simulink library "NMEA"  (R2024a)
settings: Solver=VariableStepAuto  StartTime=0.0  StopTime=10.0  RelTol=1e-3
libraries: $bdroot x44, simulink x21, simulink_extras x17, etargetslib x14
(part 3 of 4)

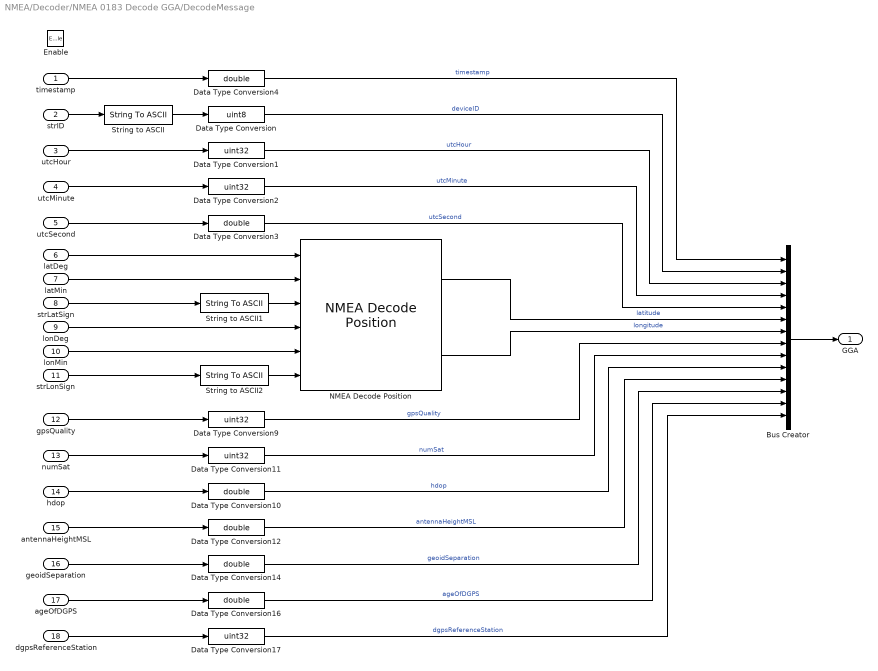
== system NMEA/Decoder/NMEA 0183 Decode GGA/DecodeMessage ==
  timestamp : Inport
  strID : Inport  Port=2
  utcHour : Inport  Port=3
  utcMinute : Inport  Port=4
  utcSecond : Inport  Port=5
  latDeg : Inport  Port=6
  latMin : Inport  Port=7
  strLatSign : Inport  Port=8
  lonDeg : Inport  Port=9
  lonMin : Inport  Port=10
  strLonSign : Inport  Port=11
  gpsQuality : Inport  Port=12
  numSat : Inport  Port=13
  hdop : Inport  Port=14
  antennaHeightMSL : Inport  Port=15
  geoidSeparation : Inport  Port=16
  ageOfDGPS : Inport  Port=17
  dgpsReferenceStation : Inport  Port=18
  Enable : EnablePort
  Bus Creator : BusCreator  Inputs=14
  Data Type Conversion : DataTypeConversion  OutDataTypeStr=uint8  SaturateOnIntegerOverflow=off  RndMeth=Floor
  Data Type Conversion{1..2,9,11,17} (5 alike) : DataTypeConversion  OutDataTypeStr=uint32  SaturateOnIntegerOverflow=off  RndMeth=Floor
  Data Type Conversion{3..4,10,12,14,16} (6 alike) : DataTypeConversion  OutDataTypeStr=double  SaturateOnIntegerOverflow=off  RndMeth=Floor
  NMEA Decode Position : $bdroot/Details/NMEA Decode Position
  String to ASCII : StringToASCII  OutputVectorSize=2
  String to ASCII1 : StringToASCII  OutputVectorSize=1
  String to ASCII2 : StringToASCII  OutputVectorSize=1
  GGA : Outport
  wires:
  Bus Creator/1 -> GGA/1
  timestamp/1 -> Data Type Conversion4/1
  strID/1 -> String to ASCII/1
  String to ASCII/1 -> Data Type Conversion/1
  Data Type Conversion/1 -> Bus Creator/2  "deviceID"
  utcHour/1 -> Data Type Conversion1/1
  utcMinute/1 -> Data Type Conversion2/1
  utcSecond/1 -> Data Type Conversion3/1
  Data Type Conversion1/1 -> Bus Creator/3  "utcHour"
  Data Type Conversion2/1 -> Bus Creator/4  "utcMinute"
  Data Type Conversion3/1 -> Bus Creator/5  "utcSecond"
  Data Type Conversion4/1 -> Bus Creator/1  "timestamp"
  gpsQuality/1 -> Data Type Conversion9/1
  numSat/1 -> Data Type Conversion11/1
  hdop/1 -> Data Type Conversion10/1
  antennaHeightMSL/1 -> Data Type Conversion12/1
  geoidSeparation/1 -> Data Type Conversion14/1
  ageOfDGPS/1 -> Data Type Conversion16/1
  dgpsReferenceStation/1 -> Data Type Conversion17/1
  Data Type Conversion9/1 -> Bus Creator/8  "gpsQuality"
  Data Type Conversion11/1 -> Bus Creator/9  "numSat"
  Data Type Conversion10/1 -> Bus Creator/10  "hdop"
  Data Type Conversion12/1 -> Bus Creator/11  "antennaHeightMSL"
  Data Type Conversion14/1 -> Bus Creator/12  "geoidSeparation"
  Data Type Conversion16/1 -> Bus Creator/13  "ageOfDGPS"
  Data Type Conversion17/1 -> Bus Creator/14  "dgpsReferenceStation"
  strLonSign/1 -> String to ASCII2/1
  String to ASCII1/1 -> NMEA Decode Position/3
  strLatSign/1 -> String to ASCII1/1
  String to ASCII2/1 -> NMEA Decode Position/6
  lonMin/1 -> NMEA Decode Position/5
  lonDeg/1 -> NMEA Decode Position/4
  latMin/1 -> NMEA Decode Position/2
  latDeg/1 -> NMEA Decode Position/1
  NMEA Decode Position/2 -> Bus Creator/7  "longitude"
  NMEA Decode Position/1 -> Bus Creator/6  "latitude"

== system NMEA/Decoder/NMEA 0183 Decode HDT/DecodeMessage ==
  timestamp : Inport
  strID : Inport  Port=2
  trueHeading : Inport  Port=3
  Enable : EnablePort
  Bus Creator : BusCreator  Inputs=3
  Data Type Conversion : DataTypeConversion  OutDataTypeStr=uint8  SaturateOnIntegerOverflow=off  RndMeth=Floor
  Data Type Conversion1 : DataTypeConversion  OutDataTypeStr=double  SaturateOnIntegerOverflow=off  RndMeth=Floor
  Data Type Conversion4 : DataTypeConversion  OutDataTypeStr=double  SaturateOnIntegerOverflow=off  RndMeth=Floor
  Degrees to Radians : simulink_extras/Transformations/Degrees to Radians
  Ensure Symmetrical Angle : $bdroot/Details/Ensure Symmetrical Angle
  String to ASCII : StringToASCII  OutputVectorSize=2
  HDT : Outport
  wires:
  Bus Creator/1 -> HDT/1
  Data Type Conversion/1 -> Bus Creator/2  "deviceID"
  Data Type Conversion4/1 -> Bus Creator/1  "timestamp"
  timestamp/1 -> Data Type Conversion4/1
  strID/1 -> String to ASCII/1
  String to ASCII/1 -> Data Type Conversion/1
  trueHeading/1 -> Data Type Conversion1/1
  Data Type Conversion1/1 -> Degrees to Radians/1
  Ensure Symmetrical Angle/1 -> Bus Creator/3  "trueHeading"
  Degrees to Radians/1 -> Ensure Symmetrical Angle/1

== system NMEA/Decoder/NMEA 0183 Decode MDA/DecodeMessage ==
  timestamp : Inport
  strID : Inport  Port=2
  pressureBar : Inport  Port=3
  airTemperatureC : Inport  Port=4
  Enable : EnablePort
  BarToPascal : Gain  Gain=1e5
  Bus Creator : BusCreator  Inputs=4
  String to ASCII : StringToASCII  OutputVectorSize=2
  MDA : Outport
  wires:
  strID/1 -> String to ASCII/1
  pressureBar/1 -> BarToPascal/1
  timestamp/1 -> Bus Creator/1  "timestamp"
  String to ASCII/1 -> Bus Creator/2  "deviceID"
  BarToPascal/1 -> Bus Creator/3  "pressure"
  airTemperatureC/1 -> Bus Creator/4  "airTemperature"
  Bus Creator/1 -> MDA/1

== system NMEA/Decoder/NMEA 0183 Decode MWV/DecodeMessage ==
  timestamp : Inport
  strID : Inport  Port=2
  windAngle : Inport  Port=3
  strWindAngleReference : Inport  Port=4
  windSpeed : Inport  Port=5
  strWindSpeedUnit : Inport  Port=6
  strStatus : Inport  Port=7
  Enable : EnablePort
  Bus Creator : BusCreator  Inputs=6
  Data Type Conversion{,2..3,5} (4 alike) : DataTypeConversion  OutDataTypeStr=uint8  SaturateOnIntegerOverflow=off  RndMeth=Floor
  Data Type Conversion1 : DataTypeConversion  OutDataTypeStr=double  SaturateOnIntegerOverflow=off  RndMeth=Floor
  Data Type Conversion11 : DataTypeConversion  OutDataTypeStr=double  SaturateOnIntegerOverflow=off  RndMeth=Floor
  Data Type Conversion4 : DataTypeConversion  OutDataTypeStr=double  SaturateOnIntegerOverflow=off  RndMeth=Floor
  Degrees to Radians : simulink_extras/Transformations/Degrees to Radians
  Ensure Symmetrical Angle : $bdroot/Details/Ensure Symmetrical Angle
  MATLAB Function : MATLAB Function  TreatAsAtomicUnit=on
  String to ASCII : StringToASCII  OutputVectorSize=2
  String to ASCII1 : StringToASCII  OutputVectorSize=1
  String to ASCII2 : StringToASCII  OutputVectorSize=1
  String to ASCII3 : StringToASCII  OutputVectorSize=1
  MWV : Outport
  wires:
  Bus Creator/1 -> MWV/1
  timestamp/1 -> Data Type Conversion4/1
  strID/1 -> String to ASCII/1
  String to ASCII/1 -> Data Type Conversion/1
  Data Type Conversion/1 -> Bus Creator/2  "deviceID"
  Data Type Conversion4/1 -> Bus Creator/1  "timestamp"
  windAngle/1 -> Data Type Conversion11/1
  windSpeed/1 -> Data Type Conversion1/1
  strWindAngleReference/1 -> String to ASCII1/1
  strWindSpeedUnit/1 -> String to ASCII2/1
  strStatus/1 -> String to ASCII3/1
  String to ASCII1/1 -> Data Type Conversion2/1
  String to ASCII2/1 -> Data Type Conversion3/1
  String to ASCII3/1 -> Data Type Conversion5/1
  Data Type Conversion11/1 -> Degrees to Radians/1
  Degrees to Radians/1 -> Ensure Symmetrical Angle/1
  Ensure Symmetrical Angle/1 -> Bus Creator/3  "windAngle"
  Data Type Conversion2/1 -> Bus Creator/4  "windAngleReference"
  Data Type Conversion1/1 -> MATLAB Function/1(windSpeedValue)
  Data Type Conversion3/1 -> MATLAB Function/2(windSpeedUnit)
  MATLAB Function/1(windSpeed) -> Bus Creator/5  "windSpeed"
  Data Type Conversion5/1 -> Bus Creator/6  "status"

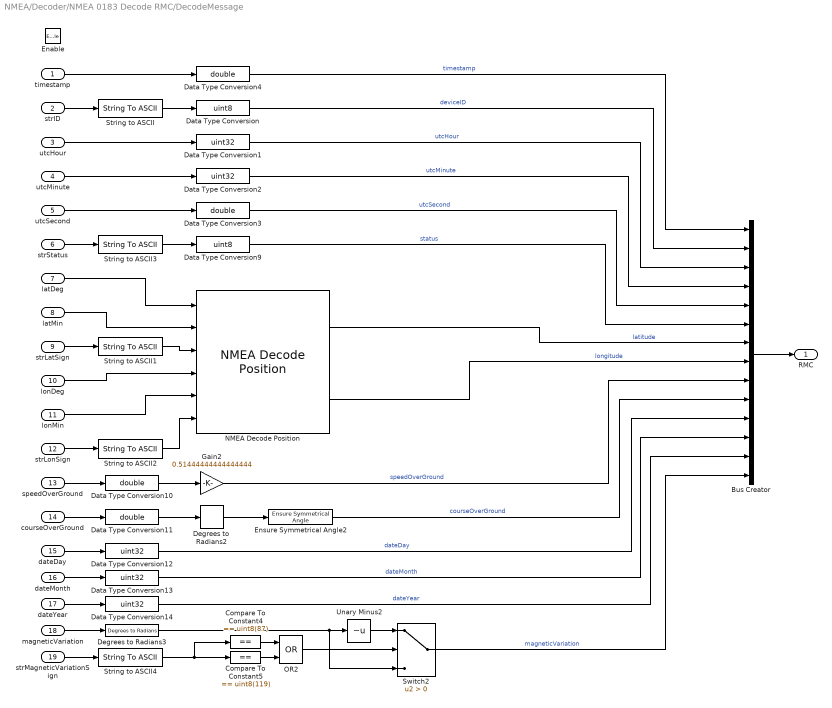
== system NMEA/Decoder/NMEA 0183 Decode RMC/DecodeMessage ==
  timestamp : Inport
  strID : Inport  Port=2
  utcHour : Inport  Port=3
  utcMinute : Inport  Port=4
  utcSecond : Inport  Port=5
  strStatus : Inport  Port=6
  latDeg : Inport  Port=7
  latMin : Inport  Port=8
  strLatSign : Inport  Port=9
  lonDeg : Inport  Port=10
  lonMin : Inport  Port=11
  strLonSign : Inport  Port=12
  speedOverGround : Inport  Port=13
  courseOverGround : Inport  Port=14
  dateDay : Inport  Port=15
  dateMonth : Inport  Port=16
  dateYear : Inport  Port=17
  magneticVariation : Inport  Port=18
  strMagneticVariationSign : Inport  Port=19
  Enable : EnablePort
  Bus Creator : BusCreator  Inputs=14
  Compare To Constant4 : simulink/Logic and Bit Operations/Compare To Constant  relop===  const=uint8(87)  OutDataTypeStr=boolean
  Compare To Constant5 : simulink/Logic and Bit Operations/Compare To Constant  relop===  const=uint8(119)  OutDataTypeStr=boolean
  Data Type Conversion : DataTypeConversion  OutDataTypeStr=uint8  SaturateOnIntegerOverflow=off  RndMeth=Floor
  Data Type Conversion{1..2,12..14} (5 alike) : DataTypeConversion  OutDataTypeStr=uint32  SaturateOnIntegerOverflow=off  RndMeth=Floor
  Data Type Conversion{3..4,10..11} (4 alike) : DataTypeConversion  OutDataTypeStr=double  SaturateOnIntegerOverflow=off  RndMeth=Floor
  Data Type Conversion9 : DataTypeConversion  OutDataTypeStr=uint8  SaturateOnIntegerOverflow=off  RndMeth=Floor
  Degrees to Radians2 : simulink_extras/Transformations/Degrees to Radians
  Degrees to Radians3 : simulink_extras/Transformations/Degrees to Radians
  Ensure Symmetrical Angle2 : $bdroot/Details/Ensure Symmetrical Angle
  Gain2 : Gain  Gain=0.51444444444444444
  NMEA Decode Position : $bdroot/Details/NMEA Decode Position
  OR2 : Logic  Operator=OR  AllPortsSameDT=off  OutDataTypeStr=boolean
  String to ASCII : StringToASCII  OutputVectorSize=2
  String to ASCII{1..4} (4 alike) : StringToASCII  OutputVectorSize=1
  Switch2 : Switch  Criteria=u2 > Threshold  SaturateOnIntegerOverflow=off  InputSameDT=off
  Unary Minus2 : UnaryMinus
  RMC : Outport
  wires:
  NMEA Decode Position/2 -> Bus Creator/8  "longitude"
  strLonSign/1 -> String to ASCII2/1
  NMEA Decode Position/1 -> Bus Creator/7  "latitude"
  strLatSign/1 -> String to ASCII1/1
  Data Type Conversion4/1 -> Bus Creator/1  "timestamp"
  Data Type Conversion3/1 -> Bus Creator/5  "utcSecond"
  Data Type Conversion2/1 -> Bus Creator/4  "utcMinute"
  Data Type Conversion1/1 -> Bus Creator/3  "utcHour"
  utcSecond/1 -> Data Type Conversion3/1
  utcMinute/1 -> Data Type Conversion2/1
  utcHour/1 -> Data Type Conversion1/1
  Data Type Conversion/1 -> Bus Creator/2  "deviceID"
  String to ASCII/1 -> Data Type Conversion/1
  strID/1 -> String to ASCII/1
  timestamp/1 -> Data Type Conversion4/1
  Bus Creator/1 -> RMC/1
  String to ASCII3/1 -> Data Type Conversion9/1
  Data Type Conversion9/1 -> Bus Creator/6  "status"
  strStatus/1 -> String to ASCII3/1
  Data Type Conversion10/1 -> Gain2/1
  speedOverGround/1 -> Data Type Conversion10/1
  Gain2/1 -> Bus Creator/9  "speedOverGround"
  courseOverGround/1 -> Data Type Conversion11/1
  Data Type Conversion11/1 -> Degrees to Radians2/1
  Degrees to Radians2/1 -> Ensure Symmetrical Angle2/1
  Ensure Symmetrical Angle2/1 -> Bus Creator/10  "courseOverGround"
  dateDay/1 -> Data Type Conversion12/1
  Data Type Conversion12/1 -> Bus Creator/11  "dateDay"
  dateMonth/1 -> Data Type Conversion13/1
  dateYear/1 -> Data Type Conversion14/1
  Data Type Conversion13/1 -> Bus Creator/12  "dateMonth"
  Data Type Conversion14/1 -> Bus Creator/13  "dateYear"
  strMagneticVariationSign/1 -> String to ASCII4/1
  Unary Minus2/1 -> Switch2/1
  OR2/1 -> Switch2/2
  Compare To Constant5/1 -> OR2/2
  Compare To Constant4/1 -> OR2/1
  String to ASCII4/1 -> Compare To Constant5/1, Compare To Constant4/1
  magneticVariation/1 -> Degrees to Radians3/1
  Switch2/1 -> Bus Creator/14  "magneticVariation"
  Degrees to Radians3/1 -> Switch2/3, Unary Minus2/1
  latMin/1 -> NMEA Decode Position/2
  latDeg/1 -> NMEA Decode Position/1
  String to ASCII1/1 -> NMEA Decode Position/3
  lonDeg/1 -> NMEA Decode Position/4
  lonMin/1 -> NMEA Decode Position/5
  String to ASCII2/1 -> NMEA Decode Position/6

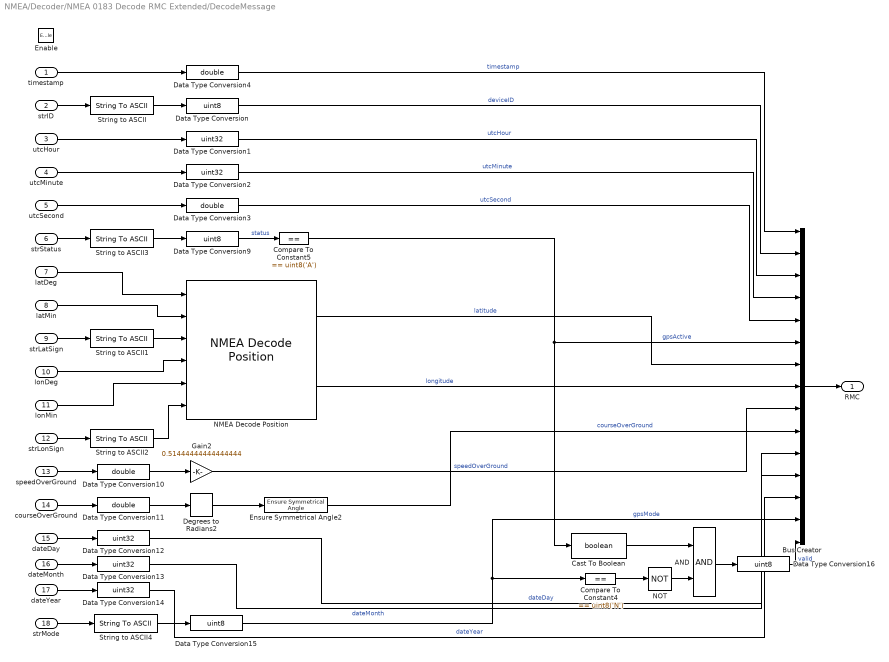
== system NMEA/Decoder/NMEA 0183 Decode RMC Extended/DecodeMessage ==
  timestamp : Inport
  strID : Inport  Port=2
  utcHour : Inport  Port=3
  utcMinute : Inport  Port=4
  utcSecond : Inport  Port=5
  strStatus : Inport  Port=6
  latDeg : Inport  Port=7
  latMin : Inport  Port=8
  strLatSign : Inport  Port=9
  lonDeg : Inport  Port=10
  lonMin : Inport  Port=11
  strLonSign : Inport  Port=12
  speedOverGround : Inport  Port=13
  courseOverGround : Inport  Port=14
  dateDay : Inport  Port=15
  dateMonth : Inport  Port=16
  dateYear : Inport  Port=17
  strMode : Inport  Port=18
  Enable : EnablePort
  AND : Logic  AllPortsSameDT=off  OutDataTypeStr=boolean
  Bus Creator : BusCreator  Inputs=15
  Cast To Boolean : DataTypeConversion  OutDataTypeStr=boolean  SaturateOnIntegerOverflow=off  RndMeth=Floor
  Compare To Constant4 : simulink/Logic and Bit Operations/Compare To Constant  relop===  const=uint8('N')  OutDataTypeStr=boolean
  Compare To Constant5 : simulink/Logic and Bit Operations/Compare To Constant  relop===  const=uint8('A')  OutDataTypeStr=uint8
  Data Type Conversion{,9,15..16} (4 alike) : DataTypeConversion  OutDataTypeStr=uint8  SaturateOnIntegerOverflow=off  RndMeth=Floor
  Data Type Conversion{1..2,12..14} (5 alike) : DataTypeConversion  OutDataTypeStr=uint32  SaturateOnIntegerOverflow=off  RndMeth=Floor
  Data Type Conversion{3..4,10..11} (4 alike) : DataTypeConversion  OutDataTypeStr=double  SaturateOnIntegerOverflow=off  RndMeth=Floor
  Degrees to Radians2 : simulink_extras/Transformations/Degrees to Radians
  Ensure Symmetrical Angle2 : $bdroot/Details/Ensure Symmetrical Angle
  Gain2 : Gain  Gain=0.51444444444444444
  NMEA Decode Position : $bdroot/Details/NMEA Decode Position
  NOT : Logic  Operator=NOT  AllPortsSameDT=off  OutDataTypeStr=boolean
  String to ASCII : StringToASCII  OutputVectorSize=2
  String to ASCII{1..4} (4 alike) : StringToASCII  OutputVectorSize=1
  RMC : Outport
  wires:
  Data Type Conversion16/1 -> Bus Creator/15  "valid"
  AND/1 -> Data Type Conversion16/1
  Cast To Boolean/1 -> AND/1
  NOT/1 -> AND/2
  Compare To Constant4/1 -> NOT/1
  Data Type Conversion14/1 -> Bus Creator/13  "dateYear"
  Data Type Conversion13/1 -> Bus Creator/12  "dateMonth"
  dateYear/1 -> Data Type Conversion14/1
  dateMonth/1 -> Data Type Conversion13/1
  Data Type Conversion12/1 -> Bus Creator/11  "dateDay"
  dateDay/1 -> Data Type Conversion12/1
  Ensure Symmetrical Angle2/1 -> Bus Creator/10  "courseOverGround"
  Degrees to Radians2/1 -> Ensure Symmetrical Angle2/1
  Data Type Conversion11/1 -> Degrees to Radians2/1
  courseOverGround/1 -> Data Type Conversion11/1
  Gain2/1 -> Bus Creator/9  "speedOverGround"
  speedOverGround/1 -> Data Type Conversion10/1
  Data Type Conversion10/1 -> Gain2/1
  strStatus/1 -> String to ASCII3/1
  Data Type Conversion9/1 -> Compare To Constant5/1  "status"
  String to ASCII3/1 -> Data Type Conversion9/1
  Bus Creator/1 -> RMC/1
  timestamp/1 -> Data Type Conversion4/1
  strID/1 -> String to ASCII/1
  String to ASCII/1 -> Data Type Conversion/1
  Data Type Conversion/1 -> Bus Creator/2  "deviceID"
  utcHour/1 -> Data Type Conversion1/1
  utcMinute/1 -> Data Type Conversion2/1
  utcSecond/1 -> Data Type Conversion3/1
  Data Type Conversion1/1 -> Bus Creator/3  "utcHour"
  Data Type Conversion2/1 -> Bus Creator/4  "utcMinute"
  Data Type Conversion3/1 -> Bus Creator/5  "utcSecond"
  Data Type Conversion4/1 -> Bus Creator/1  "timestamp"
  strLatSign/1 -> String to ASCII1/1
  strLonSign/1 -> String to ASCII2/1
  NMEA Decode Position/2 -> Bus Creator/8  "longitude"
  String to ASCII4/1 -> Data Type Conversion15/1
  strMode/1 -> String to ASCII4/1
  Data Type Conversion15/1 -> Bus Creator/14, Compare To Constant4/1  "gpsMode"
  Compare To Constant5/1 -> Bus Creator/6, Cast To Boolean/1  "gpsActive"
  latMin/1 -> NMEA Decode Position/2
  latDeg/1 -> NMEA Decode Position/1
  String to ASCII1/1 -> NMEA Decode Position/3
  lonDeg/1 -> NMEA Decode Position/4
  lonMin/1 -> NMEA Decode Position/5
  String to ASCII2/1 -> NMEA Decode Position/6
  NMEA Decode Position/1 -> Bus Creator/7  "latitude"

== system NMEA/Decoder/NMEA 0183 Decode ROT/DecodeMessage ==
  timestamp : Inport
  strID : Inport  Port=2
  rateOfTurn : Inport  Port=3
  status : Inport  Port=4
  Enable : EnablePort
  Bus Creator : BusCreator  Inputs=4
  Data Type Conversion : DataTypeConversion  OutDataTypeStr=uint8  SaturateOnIntegerOverflow=off  RndMeth=Floor
  Data Type Conversion1 : DataTypeConversion  OutDataTypeStr=double  SaturateOnIntegerOverflow=off  RndMeth=Floor
  Data Type Conversion2 : DataTypeConversion  OutDataTypeStr=uint8  SaturateOnIntegerOverflow=off  RndMeth=Floor
  Data Type Conversion4 : DataTypeConversion  OutDataTypeStr=double  SaturateOnIntegerOverflow=off  RndMeth=Floor
  Degrees to Radians : simulink_extras/Transformations/Degrees to Radians
  Gain : Gain  Gain=1/60
  String to ASCII : StringToASCII  OutputVectorSize=2
  String to ASCII1 : StringToASCII  OutputVectorSize=1
  ROT : Outport
  wires:
  Degrees to Radians/1 -> Bus Creator/3  "rateOfTurn"
  Data Type Conversion1/1 -> Gain/1
  rateOfTurn/1 -> Data Type Conversion1/1
  String to ASCII/1 -> Data Type Conversion/1
  strID/1 -> String to ASCII/1
  timestamp/1 -> Data Type Conversion4/1
  Data Type Conversion4/1 -> Bus Creator/1  "timestamp"
  Data Type Conversion/1 -> Bus Creator/2  "deviceID"
  Bus Creator/1 -> ROT/1
  status/1 -> String to ASCII1/1
  String to ASCII1/1 -> Data Type Conversion2/1
  Data Type Conversion2/1 -> Bus Creator/4  "status"
  Gain/1 -> Degrees to Radians/1

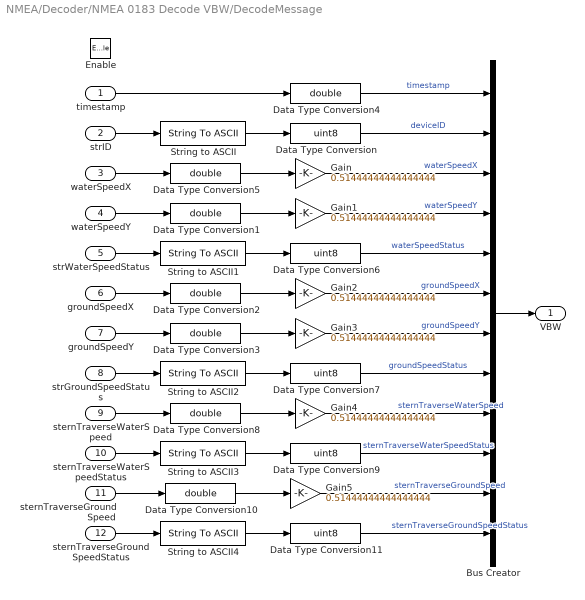
== system NMEA/Decoder/NMEA 0183 Decode VBW/DecodeMessage ==
  timestamp : Inport
  strID : Inport  Port=2
  waterSpeedX : Inport  Port=3  PortDimensions=1
  waterSpeedY : Inport  Port=4  PortDimensions=1
  strWaterSpeedStatus : Inport  Port=5
  groundSpeedX : Inport  Port=6  PortDimensions=1
  groundSpeedY : Inport  Port=7  PortDimensions=1
  strGroundSpeedStatus : Inport  Port=8
  sternTraverseWaterSpeed : Inport  Port=9
  sternTraverseWaterSpeedStatus : Inport  Port=10
  sternTraverseGroundSpeed : Inport  Port=11
  sternTraverseGroundSpeedStatus : Inport  Port=12
  Enable : EnablePort
  Bus Creator : BusCreator  Inputs=12
  Data Type Conversion{,6..7,9,11} (5 alike) : DataTypeConversion  OutDataTypeStr=uint8  SaturateOnIntegerOverflow=off  RndMeth=Floor
  Data Type Conversion{1..5,8,10} (7 alike) : DataTypeConversion  OutDataTypeStr=double  SaturateOnIntegerOverflow=off  RndMeth=Floor
  Gain{,1..5} (6 alike) : Gain  Gain=0.51444444444444444
  String to ASCII : StringToASCII  OutputVectorSize=2
  String to ASCII{1..4} (4 alike) : StringToASCII  OutputVectorSize=1
  VBW : Outport
  wires:
  String to ASCII/1 -> Data Type Conversion/1
  strID/1 -> String to ASCII/1
  timestamp/1 -> Data Type Conversion4/1
  Data Type Conversion4/1 -> Bus Creator/1  "timestamp"
  Data Type Conversion/1 -> Bus Creator/2  "deviceID"
  waterSpeedX/1 -> Data Type Conversion5/1
  waterSpeedY/1 -> Data Type Conversion1/1
  groundSpeedX/1 -> Data Type Conversion2/1
  groundSpeedY/1 -> Data Type Conversion3/1
  Data Type Conversion5/1 -> Gain/1
  Data Type Conversion1/1 -> Gain1/1
  Data Type Conversion2/1 -> Gain2/1
  Data Type Conversion3/1 -> Gain3/1
  Gain/1 -> Bus Creator/3  "waterSpeedX"
  Gain1/1 -> Bus Creator/4  "waterSpeedY"
  Gain2/1 -> Bus Creator/6  "groundSpeedX"
  strWaterSpeedStatus/1 -> String to ASCII1/1
  String to ASCII1/1 -> Data Type Conversion6/1
  Data Type Conversion6/1 -> Bus Creator/5  "waterSpeedStatus"
  Data Type Conversion7/1 -> Bus Creator/8  "groundSpeedStatus"
  String to ASCII2/1 -> Data Type Conversion7/1
  strGroundSpeedStatus/1 -> String to ASCII2/1
  Gain3/1 -> Bus Creator/7  "groundSpeedY"
  Bus Creator/1 -> VBW/1
  sternTraverseWaterSpeed/1 -> Data Type Conversion8/1
  Data Type Conversion8/1 -> Gain4/1
  Gain4/1 -> Bus Creator/9  "sternTraverseWaterSpeed"
  sternTraverseWaterSpeedStatus/1 -> String to ASCII3/1
  String to ASCII3/1 -> Data Type Conversion9/1
  Data Type Conversion9/1 -> Bus Creator/10  "sternTraverseWaterSpeedStatus"
  sternTraverseGroundSpeed/1 -> Data Type Conversion10/1
  sternTraverseGroundSpeedStatus/1 -> String to ASCII4/1
  Data Type Conversion10/1 -> Gain5/1
  String to ASCII4/1 -> Data Type Conversion11/1
  Gain5/1 -> Bus Creator/11  "sternTraverseGroundSpeed"
  Data Type Conversion11/1 -> Bus Creator/12  "sternTraverseGroundSpeedStatus"

== system NMEA/Decoder/NMEA 0183 Decode VTG/DecodeMessage ==
  timestamp : Inport
  strID : Inport  Port=2
  trackMadeGoodTrue : Inport  Port=3
  trackMadeGoodMagnetic : Inport  Port=4
  speedOverGround1 : Inport  Port=5
  speedOverGround2 : Inport  Port=6
  mode : Inport  Port=7
  Enable : EnablePort
  Bus Creator : BusCreator  Inputs=7
  Data Type Conversion : DataTypeConversion  OutDataTypeStr=uint8  SaturateOnIntegerOverflow=off  RndMeth=Floor
  Data Type Conversion{1..4,11} (5 alike) : DataTypeConversion  OutDataTypeStr=double  SaturateOnIntegerOverflow=off  RndMeth=Floor
  Data Type Conversion5 : DataTypeConversion  OutDataTypeStr=uint8  SaturateOnIntegerOverflow=off  RndMeth=Floor
  Degrees to Radians1 : simulink_extras/Transformations/Degrees to Radians
  Degrees to Radians2 : simulink_extras/Transformations/Degrees to Radians
  Ensure Symmetrical Angle : $bdroot/Details/Ensure Symmetrical Angle
  Ensure Symmetrical Angle1 : $bdroot/Details/Ensure Symmetrical Angle
  KPHToMPS : Gain  Gain=1/3.6
  KnotsToMPS : Gain  Gain=0.51444444444444444
  String to ASCII : StringToASCII  OutputVectorSize=2
  String to ASCII1 : StringToASCII  OutputVectorSize=1
  VTG : Outport
  wires:
  Degrees to Radians2/1 -> Ensure Symmetrical Angle/1
  Data Type Conversion11/1 -> Degrees to Radians2/1
  Bus Creator/1 -> VTG/1
  timestamp/1 -> Data Type Conversion4/1
  strID/1 -> String to ASCII/1
  String to ASCII/1 -> Data Type Conversion/1
  Data Type Conversion/1 -> Bus Creator/2  "deviceID"
  Data Type Conversion4/1 -> Bus Creator/1  "timestamp"
  trackMadeGoodTrue/1 -> Data Type Conversion11/1
  trackMadeGoodMagnetic/1 -> Data Type Conversion1/1
  Data Type Conversion1/1 -> Degrees to Radians1/1
  Degrees to Radians1/1 -> Ensure Symmetrical Angle1/1
  speedOverGround1/1 -> Data Type Conversion2/1
  Data Type Conversion2/1 -> KnotsToMPS/1
  speedOverGround2/1 -> Data Type Conversion3/1
  Data Type Conversion3/1 -> KPHToMPS/1
  Ensure Symmetrical Angle/1 -> Bus Creator/3  "trackMadeGoodTrue"
  Ensure Symmetrical Angle1/1 -> Bus Creator/4  "trackMadeGoodMagnetic"
  KnotsToMPS/1 -> Bus Creator/5  "speedOverGround1"
  KPHToMPS/1 -> Bus Creator/6  "speedOverGround2"
  mode/1 -> String to ASCII1/1
  String to ASCII1/1 -> Data Type Conversion5/1
  Data Type Conversion5/1 -> Bus Creator/7  "mode"

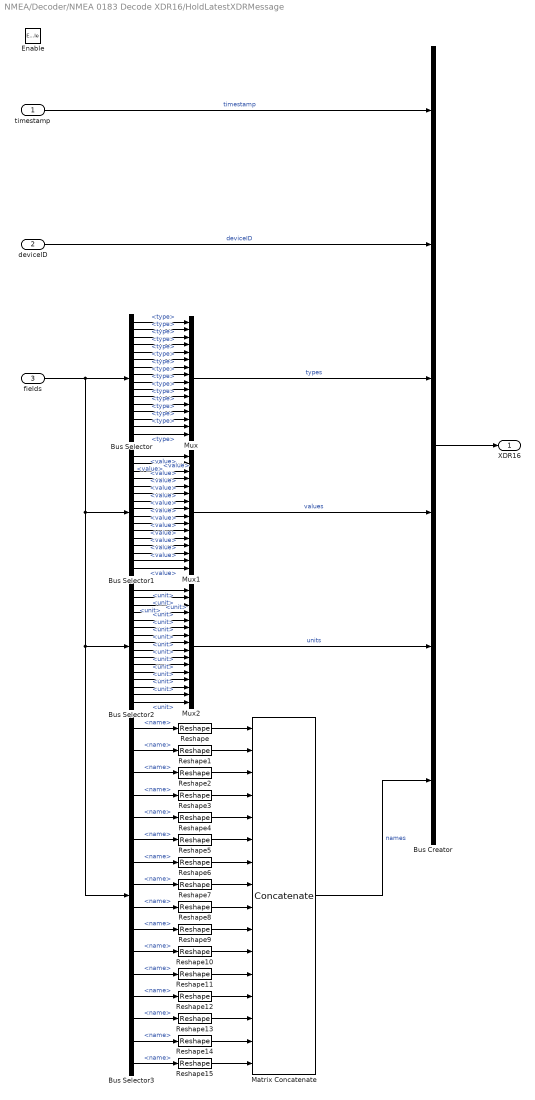
== system NMEA/Decoder/NMEA 0183 Decode XDR16/HoldLatestXDRMessage ==
  timestamp : Inport
  deviceID : Inport  Port=2
  fields : Inport  Port=3
  Enable : EnablePort
  Bus Creator : BusCreator  Inputs=6
  Bus Selector : BusSelector  OutputSignals=field1.type,field2.type,field3.type,field4.type,field5.type,field6.type,field7.type,field8.type,field9.type,field10.type,field11.type,field12.type,field13.type,field14.type,field15.type,field16.type
  Bus Selector1 : BusSelector  OutputSignals=field1.value,field2.value,field3.value,field4.value,field5.value,field6.value,field7.value,field8.value,field9.value,field10.value,field11.value,field12.value,field13.value,field14.value,field15.value,field16.value
  Bus Selector2 : BusSelector  OutputSignals=field1.unit,field2.unit,field3.unit,field4.unit,field5.unit,field6.unit,field7.unit,field8.unit,field9.unit,field10.unit,field11.unit,field12.unit,field13.unit,field14.unit,field15.unit,field16.unit
  Bus Selector3 : BusSelector  OutputSignals=field1.name,field2.name,field3.name,field4.name,field5.name,field6.name,field7.name,field8.name,field9.name,field10.name,field11.name,field12.name,field13.name,field14.name,field15.name,field16.name
  Matrix Concatenate : Concatenate  NumInputs=16  Mode=Multidimensional array  ConcatenateDimension=2
  Mux : Mux  Inputs=16
  Mux1 : Mux  Inputs=16
  Mux2 : Mux  Inputs=16
  Reshape{,1..15} (16 alike) : Reshape  OutputDimensionality=Customize  OutputDimensions=[4,1]
  XDR16 : Outport
  wires:
  Bus Selector/15 -> Mux/15  "<type>"
  Bus Selector1/5 -> Mux1/5  "<value>"
  Reshape10/1 -> Matrix Concatenate/11
  Bus Selector1/4 -> Mux1/4  "<value>"
  Bus Selector/16 -> Mux/16  "<type>"
  Reshape1/1 -> Matrix Concatenate/2
  Bus Selector3/16 -> Reshape15/1  "<name>"
  Bus Selector3/14 -> Reshape13/1  "<name>"
  Bus Selector3/5 -> Reshape4/1  "<name>"
  Bus Selector2/16 -> Mux2/16  "<unit>"
  Bus Selector3/2 -> Reshape1/1  "<name>"
  Bus Selector/4 -> Mux/4  "<type>"
  Bus Selector1/1 -> Mux1/1  "<value>"
  Reshape5/1 -> Matrix Concatenate/6
  Bus Selector/14 -> Mux/14  "<type>"
  Reshape9/1 -> Matrix Concatenate/10
  Bus Selector1/6 -> Mux1/6  "<value>"
  Bus Selector/9 -> Mux/9  "<type>"
  Reshape2/1 -> Matrix Concatenate/3
  Bus Selector1/7 -> Mux1/7  "<value>"
  Bus Selector/10 -> Mux/10  "<type>"
  Bus Selector3/7 -> Reshape6/1  "<name>"
  Bus Selector1/8 -> Mux1/8  "<value>"
  Bus Selector2/8 -> Mux2/8  "<unit>"
  Bus Selector/1 -> Mux/1  "<type>"
  Bus Selector2/11 -> Mux2/11  "<unit>"
  Bus Selector1/15 -> Mux1/15  "<value>"
  Bus Selector/5 -> Mux/5  "<type>"
  Bus Selector1/2 -> Mux1/2  "<value>"
  Bus Selector1/16 -> Mux1/16  "<value>"
  Bus Selector3/8 -> Reshape7/1  "<name>"
  Bus Selector2/1 -> Mux2/1  "<unit>"
  Bus Selector1/3 -> Mux1/3  "<value>"
  Bus Selector2/12 -> Mux2/12  "<unit>"
  Reshape13/1 -> Matrix Concatenate/14
  Bus Selector3/9 -> Reshape8/1  "<name>"
  Bus Selector3/10 -> Reshape9/1  "<name>"
  Reshape15/1 -> Matrix Concatenate/16
  Reshape14/1 -> Matrix Concatenate/15
  Bus Selector2/6 -> Mux2/6  "<unit>"
  Bus Selector3/15 -> Reshape14/1  "<name>"
  Bus Selector2/2 -> Mux2/2  "<unit>"
  Bus Selector3/11 -> Reshape10/1  "<name>"
  Bus Selector3/13 -> Reshape12/1  "<name>"
  Bus Selector2/15 -> Mux2/15  "<unit>"
  Reshape/1 -> Matrix Concatenate/1
  fields/1 -> Bus Selector3/1, Bus Selector2/1, Bus Selector1/1, Bus Selector/1
  Reshape8/1 -> Matrix Concatenate/9
  Bus Selector3/3 -> Reshape2/1  "<name>"
  Reshape12/1 -> Matrix Concatenate/13
  Bus Selector1/14 -> Mux1/14  "<value>"
  Bus Selector2/9 -> Mux2/9  "<unit>"
  Bus Selector2/10 -> Mux2/10  "<unit>"
  Bus Selector1/13 -> Mux1/13  "<value>"
  Bus Selector3/6 -> Reshape5/1  "<name>"
  Bus Selector2/5 -> Mux2/5  "<unit>"
  Bus Selector2/3 -> Mux2/3  "<unit>"
  Reshape3/1 -> Matrix Concatenate/4
  Reshape11/1 -> Matrix Concatenate/12
  Bus Selector2/4 -> Mux2/4  "<unit>"
  Bus Selector/13 -> Mux/13  "<type>"
  Bus Selector1/9 -> Mux1/9  "<value>"
  Reshape4/1 -> Matrix Concatenate/5
  Bus Selector/3 -> Mux/3  "<type>"
  Bus Selector1/11 -> Mux1/11  "<value>"
  Bus Selector3/12 -> Reshape11/1  "<name>"
  Reshape6/1 -> Matrix Concatenate/7
  Bus Selector2/14 -> Mux2/14  "<unit>"
  Bus Selector1/12 -> Mux1/12  "<value>"
  Bus Selector3/4 -> Reshape3/1  "<name>"
  Bus Selector/6 -> Mux/6  "<type>"
  Bus Selector2/7 -> Mux2/7  "<unit>"
  Bus Selector/2 -> Mux/2  "<type>"
  Bus Selector1/10 -> Mux1/10  "<value>"
  Bus Selector2/13 -> Mux2/13  "<unit>"
  Bus Selector/8 -> Mux/8  "<type>"
  Reshape7/1 -> Matrix Concatenate/8
  Bus Selector3/1 -> Reshape/1  "<name>"
  Bus Selector/11 -> Mux/11  "<type>"
  Bus Selector/12 -> Mux/12  "<type>"
  Bus Selector/7 -> Mux/7  "<type>"
  timestamp/1 -> Bus Creator/1  "timestamp"
  deviceID/1 -> Bus Creator/2  "deviceID"
  Mux/1 -> Bus Creator/3  "types"
  Mux1/1 -> Bus Creator/4  "values"
  Mux2/1 -> Bus Creator/5  "units"
  Matrix Concatenate/1 -> Bus Creator/6  "names"
  Bus Creator/1 -> XDR16/1

== system NMEA/Decoder/NMEA 0183 Decode ZDA/DecodeMessage ==
  timestamp : Inport
  strID : Inport  Port=2
  utcHour : Inport  Port=3
  utcMinute : Inport  Port=4
  utcSecond : Inport  Port=5
  utcDay : Inport  Port=6
  utcMonth : Inport  Port=7
  utcYear : Inport  Port=8
  localTimeZoneOffsetFromGMTHour : Inport  Port=9
  localTimeZoneOffsetFromGMTMinute : Inport  Port=10
  Enable : EnablePort
  Bus Creator : BusCreator  Inputs=10
  Data Type Conversion : DataTypeConversion  OutDataTypeStr=uint8  SaturateOnIntegerOverflow=off  RndMeth=Floor
  Data Type Conversion{1..2,5..9} (7 alike) : DataTypeConversion  OutDataTypeStr=uint32  SaturateOnIntegerOverflow=off  RndMeth=Floor
  Data Type Conversion3 : DataTypeConversion  OutDataTypeStr=double  SaturateOnIntegerOverflow=off  RndMeth=Floor
  Data Type Conversion4 : DataTypeConversion  OutDataTypeStr=double  SaturateOnIntegerOverflow=off  RndMeth=Floor
  String to ASCII : StringToASCII  OutputVectorSize=2
  ZDA : Outport
  wires:
  Data Type Conversion4/1 -> Bus Creator/1  "timestamp"
  Data Type Conversion3/1 -> Bus Creator/5  "utcSecond"
  Data Type Conversion2/1 -> Bus Creator/4  "utcMinute"
  Data Type Conversion1/1 -> Bus Creator/3  "utcHour"
  utcSecond/1 -> Data Type Conversion3/1
  utcMinute/1 -> Data Type Conversion2/1
  utcHour/1 -> Data Type Conversion1/1
  Data Type Conversion/1 -> Bus Creator/2  "deviceID"
  String to ASCII/1 -> Data Type Conversion/1
  strID/1 -> String to ASCII/1
  timestamp/1 -> Data Type Conversion4/1
  Bus Creator/1 -> ZDA/1
  utcDay/1 -> Data Type Conversion5/1
  utcMonth/1 -> Data Type Conversion6/1
  utcYear/1 -> Data Type Conversion7/1
  Data Type Conversion5/1 -> Bus Creator/6  "utcDay"
  Data Type Conversion6/1 -> Bus Creator/7  "utcMonth"
  Data Type Conversion7/1 -> Bus Creator/8  "utcYear"
  localTimeZoneOffsetFromGMTHour/1 -> Data Type Conversion8/1
  localTimeZoneOffsetFromGMTMinute/1 -> Data Type Conversion9/1
  Data Type Conversion8/1 -> Bus Creator/9  "localTimeZoneOffsetFromGMTHour"
  Data Type Conversion9/1 -> Bus Creator/10  "localTimeZoneOffsetFromGMTMinute"

== matlab function NMEA/Details/NMEA Checksum Test/MATLAB Function ==
  data: bytes input; isCorrect output; len input
function isCorrect = NMEAChecksumIsCorrect(bytes, len)
    len = uint32(min(len, length(bytes)));
    isCorrect = false;
    cs = uint8(0);
    mode = uint32(0);
    for i = uint32(1):len
        switch(mode)
            case uint32(0)
                if(uint8('$') == bytes(i))
                    mode = uint32(1);
                end
            case uint32(1)
                if(uint8('*') == bytes(i))
                    if((i + uint32(2)) <= len)
                        isCorrect = (cs == uint8(hex2dec([char(bytes(i + uint32(1))) char(bytes(i + uint32(2)))])));
                    end
                    break;
                end
                cs = bitxor(cs, bytes(i));
        end
    end
end

== matlab function NMEA/Details/NMEA Fill Empty Fields/MATLAB Function ==
  data: bytesIn input; bytesOut output; lengthIn input; lengthOut output
function [bytesOut, lengthOut] = FillEmptyFields(bytesIn, lengthIn)
    bytesOut = bytesIn;
    lengthOut = lengthIn;
    N = length(bytesIn);
    lengthIn = min(lengthIn, N);
    iOut = 2;
    for i = 2:lengthIn
        if(((uint8(',') == bytesIn(i)) && (uint8(',') == bytesIn(i - 1))) || ((uint8('*') == bytesIn(i)) && (uint8(',') == bytesIn(i - 1))))
            bytesOut(iOut) = '0';
            iOut = iOut + 1;
            if(iOut > N), break; end
            bytesOut(iOut) = bytesIn(i);
            iOut = iOut + 1;
            lengthOut = lengthOut + 1;
            if(iOut > N), break; end
        else
            bytesOut(iOut) = bytesIn(i);
            iOut = iOut + 1;
            if(iOut > N), break; end
        end
    end
end

== matlab function NMEA/Details/NMEA XDR16 Get Value Of Transducer/MATLAB Function ==
  data: transducerName input uint8 size=4; value output double size=1; typesXDR input uint8; valuesXDR input double; unitsXDR input uint8; namesXDR input uint8; found output boolean size=1
function [value,found] = GetValueOfTransducer(transducerName, typesXDR, valuesXDR, unitsXDR, namesXDR)
    % Get number of fields
    N = length(typesXDR);
    N = min(N, length(valuesXDR));
    N = min(N, length(unitsXDR));
    N = min(N, size(namesXDR,2));

    % Fallback output
    value = 0;
    found = false;

    % Go through all fields and find the first name that matches the transducer name
    for n = 1:N
        if((transducerName(1) == namesXDR(1,n)) && (transducerName(2) == namesXDR(2,n)) && (transducerName(3) == namesXDR(3,n)) && (transducerName(4) == namesXDR(4,n)))
            scaleToSI = 1.0;
            switch(unitsXDR(n))
                case uint8('B') % Bar: convert to Pa
                    scaleToSI = 1e5;
                case uint8('C') % Celsius: no scale needed
                    scaleToSI = 1.0;
                case uint8('D') % Degrees: convert to rad
                    scaleToSI = deg2rad(1.0);
                case uint8('M') % Meter: no scale needed
                    scaleToSI = 1.0;
                case uint8('N') % Newton: no scale needed
                    scaleToSI = 1.0;
                case uint8('P') % Percent: convert to 1
                    scaleToSI = 0.01;
            end
            value = valuesXDR(n) * scaleToSI;
            found = true;
            break;
        end
    end
end

== matlab function NMEA/Details/NMEA Encode Position/EncodePosition ==
  data: lat input; latDeg output; lon input; latMin output; latChar output; lonDeg output; lonMin output; lonChar output
function [latDeg, latMin, latChar, lonDeg, lonMin, lonChar] = EncodePosition(lat, lon)
    % Ensure that both input angles are symmetric
    x = lat;
    x = x - 6.28318530717959 * fix(x * 0.159154943091895);
    lat = x + 6.28318530717959 * double(x < -3.14159265358979) - 6.28318530717959 * double(x >= 3.14159265358979);
    x = lon;
    x = x - 6.28318530717959 * fix(x * 0.159154943091895);
    lon = x + 6.28318530717959 * double(x < -3.14159265358979) - 6.28318530717959 * double(x >= 3.14159265358979);

    % Set character based on sign
    latChar = uint8('N');
    lonChar = uint8('E');
    if(lat < 0.0), latChar = uint8('S'); end
    if(lon < 0.0), lonChar = uint8('W'); end

    % Convert to deg and min
    lat = rad2deg(abs(lat));
    lon = rad2deg(abs(lon));
    latDeg = uint32(fix(lat));
    lonDeg = uint32(fix(lon));
    latMin = (lat - double(latDeg)) * 60.0;
    lonMin = (lon - double(lonDeg)) * 60.0;
end

== matlab function NMEA/Details/Ensure Symmetrical Angle/Symmetrical Angle ==
  data: x input double; y output double
function y = SymmetricalAngle(x)
    %SymmetricalAngle Convert a given angle x [rad] to an output angle y [rad] with y being in range [-pi, +pi).
    % 
    % PARAMETERS
    % x ... Input angle in radians, either scalar or n-dimensional.
    % 
    % RETURN
    % y ... Output angle in radians being in range [-pi, pi).
    pi2 = pi + pi;
    x = x - pi2 * fix(x / pi2);
    y = x + pi2 * (double(x < -pi) - double(x >= pi));
end

== matlab function NMEA/Details/Ensure Positive Angle/Positive Angle ==
  data: x input double; y output double
function y = PositiveAngle(x)
    %PositiveAngle Convert a given angle x [rad] to an output angle y [rad] with y being in range [0, +2*pi).
    % 
    % PARAMETERS
    % x ... Input angle in radians, either scalar or n-dimensional.
    % 
    % RETURN
    % y ... Output angle in radians being in range [0, +2*pi).
    pi2 = pi + pi;
    x = x - pi2 * fix(x / pi2);
    y = x + pi2 * double(x < 0.0);
end

== matlab function NMEA/NMEA 0183 Demuxer/Demuxer ==
  data: timeSource input double size=1; bytes input uint8; len input int32 size=1; messages output uint8 size=[(8+bufferSize) numMessages]; numMessages parameter size=1; bufferSize parameter int32 size=1; ignoreChecksum parameter boolean size=1; idStrings input
function messages = NMEADemuxer(timeSource, bytes, len, numMessages, bufferSize, ignoreChecksum, idStrings)
    % ~~~~~~~~~~~~~~~~~~~~~~~~~~~~~~~~~~~~~~~~~~~~~~~~~~~~~~~~~~~~~~~~~~~
    % Maintain some values across function calls
    % ~~~~~~~~~~~~~~~~~~~~~~~~~~~~~~~~~~~~~~~~~~~~~~~~~~~~~~~~~~~~~~~~~~~
    persistent buffer;
    if(isempty(buffer)), buffer = uint8(zeros(bufferSize,1)); end
    persistent idxBuffer;
    if(isempty(idxBuffer)), idxBuffer = int32(1); end
    persistent checksumMode;
    if(isempty(checksumMode)), checksumMode = int32(0); end
    persistent messageBuffer;
    if(isempty(messageBuffer)), messageBuffer = uint8(zeros(8 + bufferSize,numMessages)); end


    % ~~~~~~~~~~~~~~~~~~~~~~~~~~~~~~~~~~~~~~~~~~~~~~~~~~~~~~~~~~~~~~~~~~~
    % Build an ID table
    % ~~~~~~~~~~~~~~~~~~~~~~~~~~~~~~~~~~~~~~~~~~~~~~~~~~~~~~~~~~~~~~~~~~~
    persistent idTable;
    if(isempty(idTable))
        idTable = uint8(zeros(length(idStrings),numMessages));
        tmp = uint8(zeros(length(idStrings),1));
        idxEntry = 1;
        n = 1;
        for i = 1:length(idStrings)
            % Add byte to tmp if no comma
            if(uint8(',') ~= idStrings(i))
                tmp(n) = idStrings(i);
                n = n + 1;
            end

            % If comma or end of string, add to table if nonempty and unique
            if((uint8(',') == idStrings(i)) || (i == length(idStrings)))
                if(n > 1)
                    % Check if tmp is already in the table
                    alreadyExists = false;
                    for j = 1:(idxEntry-1)
                        if(length(idStrings) == sum(idTable(:,j) == tmp))
                            alreadyExists = true;
                            break;
                        end
                    end

                    % Add tmp to table
                    if(~alreadyExists)
                        idTable(:,idxEntry) = tmp;
                        idxEntry = idxEntry + 1;
                        if(idxEntry > numMessages)
                            break;
                        end
                    end
                end
                tmp = uint8(zeros(length(idStrings),1));
                n = 1;
            end
        end
    end


    % ~~~~~~~~~~~~~~~~~~~~~~~~~~~~~~~~~~~~~~~~~~~~~~~~~~~~~~~~~~~~~~~~~~~
    % Fill buffer with stream data
    % ~~~~~~~~~~~~~~~~~~~~~~~~~~~~~~~~~~~~~~~~~~~~~~~~~~~~~~~~~~~~~~~~~~~
    for i = int32(1):len
        % Invalid character (non-ASCII): restart buffer
        if((bytes(i) < uint8(32)) || (bytes(i) > uint8(126)))
            idxBuffer = int32(1);
            checksumMode = int32(0);
            continue;
        end

        % Start-delimiter ('$'): restart buffer with new message
        if(uint8('$') == bytes(i))
            buffer(1) = bytes(i);
            idxBuffer = int32(2);
            if(idxBuffer > bufferSize)
                idxBuffer = int32(1);
            end
            checksumMode = int32(0);
            continue;
        end

        % Start delimiter ('$') must already be in the buffer
        if(idxBuffer > int32(1))
            % Add new byte to message and update index
            buffer(idxBuffer) = bytes(i);
            idxBuffer = idxBuffer + int32(1);
            if(idxBuffer > bufferSize)
                idxBuffer = int32(1);
                checksumMode = int32(0);
                continue;
            end
            switch(checksumMode)
                case 0
                    % If '*' delimiter found: enter checksum mode
                    if(uint8('*') == bytes(i))
                        checksumMode = int32(1);
                    end
                case 1
                    % Ensure valid checksum format
                    if(~((bytes(i) >= uint8('0')) && (bytes(i) <= uint8('9')) || (bytes(i) >= uint8('A')) && (bytes(i) <= uint8('F')) || (bytes(i) >= uint8('a')) && (bytes(i) <= uint8('f'))))
                        idxBuffer = int32(1);
                        checksumMode = int32(0);
                        continue;
                    end

                    % 1st byte of checksum received: update checksum mode to 2
                    checksumMode = int32(2);
                case 2
                    % Ensure valid checksum format
                    if(~((bytes(i) >= uint8('0')) && (bytes(i) <= uint8('9')) || (bytes(i) >= uint8('A')) && (bytes(i) <= uint8('F')) || (bytes(i) >= uint8('a')) && (bytes(i) <= uint8('f'))))
                        idxBuffer = int32(1);
                        checksumMode = int32(0);
                        continue;
                    end

                    % 2nd byte of checksum received: compute and compare checksum
                    cs = uint8(0);
                    for n = int32(2):(idxBuffer - int32(4))
                        cs = bitxor(cs, buffer(n));
                    end
                    msb = char(buffer(idxBuffer - 2));
                    lsb = char(buffer(idxBuffer - 1));
                    if((cs == uint8(hex2dec([msb lsb]))) || ignoreChecksum)
                        % Go through ID table and find index of column that matches with start string of message
                        idxEntry = int32(0);
                        for e = int32(1):int32(numMessages)
                            % Check for equal entry
                            isEqual = false;
                            for n = int32(1):int32(length(idStrings))
                                % ID table entry does not contain more bytes to compare (0)
                                if(~idTable(n,e)), break; end

                                % Message has no more bytes, but ID table entry still has bytes -> not equal
                                if((n + int32(1)) >= idxBuffer)
                                    isEqual = false;
                                    break;
                                end

                                % Check bytes
                                isEqual = (buffer(n + int32(1)) == idTable(n,e));
                                if(~isEqual), break; end
                            end

                            % If entry is equal to begin of message string, save entry index and stop search
                            if(isEqual)
                                idxEntry = e;
                                break;
                            end
                        end

                        % Go on if entry index is valid
                        if(idxEntry > int32(0))
                            % Clear buffer (set zeros), add timestamp, copy read buffer to specific entry of output message buffer
                            messageBuffer(:,idxEntry) = uint8(zeros(8 + bufferSize,1));
                            messageBuffer(1:8,idxEntry) = typecast(double(timeSource),'uint8')';
                            messageBuffer(9:7+idxBuffer,idxEntry) = buffer(1:idxBuffer-1);
                        end
                    end

                    % Reset buffer to start with a new message
                    idxBuffer = int32(1);
                    checksumMode = int32(0);
            end
        end
    end

    % ~~~~~~~~~~~~~~~~~~~~~~~~~~~~~~~~~~~~~~~~~~~~~~~~~~~~~~~~~~~~~~~~~~~
    % Assign output values
    % ~~~~~~~~~~~~~~~~~~~~~~~~~~~~~~~~~~~~~~~~~~~~~~~~~~~~~~~~~~~~~~~~~~~
    messages = messageBuffer;
end

== matlab function NMEA/NMEA 0183 TAG Split/MATLAB Function ==
  data: bytes input uint8; tag_c output uint8; len input uint32 size=1; tag_d output uint8; tag_g output uint8; tag_n output uint8; tag_r output uint8; tag_s output uint8; tag_t output uint8; payloadBytes output uint8; payloadLength output uint32 size=1; ignoreChecksum parameter boolean size=1
function [tag_c,tag_d,tag_g,tag_n,tag_r,tag_s,tag_t,payloadBytes,payloadLength] = DecodeNMEA0183WithTAGBlock(bytes, len, ignoreChecksum)
    % ~~~~~~~~~~~~~~~~~~~~~~~~~~~~~~~~~~~~~~~~~~~~~~~~~~~~~~~~~~~~~~~~~~~~~~~~~~~~~~~~~~~~~~~~~~~~~~~~~~~~~~~~~~~~~~~~~~~~~~~~~
    % For now, we support TAG parameter values up to 16 characters. The following parameter codes are supported.
    % 
    % parameter code   parameter name
    % --------------   --------------
    %       c           UNIX time
    %       d           Destination Id
    %       g           Grouping
    %       n           Line count
    %       r           Relative time
    %       s           Source Id
    %       t           Text string
    % ~~~~~~~~~~~~~~~~~~~~~~~~~~~~~~~~~~~~~~~~~~~~~~~~~~~~~~~~~~~~~~~~~~~~~~~~~~~~~~~~~~~~~~~~~~~~~~~~~~~~~~~~~~~~~~~~~~~~~~~~~


    % ~~~~~~~~~~~~~~~~~~~~~~~~~~~~~~~~~~~~~~~~~~~~~~~~~~~~~~~~~~~~~~~~~~~~~~~~~~~~~~~~~~~~~~~~~~~~~~~~~~~~~~~~~~~~~~~~~~~~~~~~~
    % Default output for payload bytes
    % ~~~~~~~~~~~~~~~~~~~~~~~~~~~~~~~~~~~~~~~~~~~~~~~~~~~~~~~~~~~~~~~~~~~~~~~~~~~~~~~~~~~~~~~~~~~~~~~~~~~~~~~~~~~~~~~~~~~~~~~~~
    payloadBytes = uint8(zeros(length(bytes),1));
    payloadLength = uint32(0);

    % ~~~~~~~~~~~~~~~~~~~~~~~~~~~~~~~~~~~~~~~~~~~~~~~~~~~~~~~~~~~~~~~~~~~~~~~~~~~~~~~~~~~~~~~~~~~~~~~~~~~~~~~~~~~~~~~~~~~~~~~~~
    % Decode byte by byte
    % ~~~~~~~~~~~~~~~~~~~~~~~~~~~~~~~~~~~~~~~~~~~~~~~~~~~~~~~~~~~~~~~~~~~~~~~~~~~~~~~~~~~~~~~~~~~~~~~~~~~~~~~~~~~~~~~~~~~~~~~~~
    len = uint32(min(len, length(bytes)));
    tagBlock = uint32(0);
    TAGbuffer = uint8(zeros(16,7));
    L = uint32(1);
    tagCode = uint32(0);
    tagMode = uint32(0);
    cs = uint8(0);
    strCS = [uint8('0'), uint8('0')];
    checksumCorrect = ignoreChecksum;
    for i = uint32(1):len
        % Begin or end of TAG block: '\'
        if((tagBlock < uint32(2)) && (uint8('\') == bytes(i)))
            tagBlock = tagBlock + uint32(1);
            continue;
        end

        % Inside the TAG block
        if(uint32(1) == tagBlock)
            switch(tagMode)
                case uint32(0) % one character: parameter code
                    tagCode = uint32(0);
                    switch(bytes(i))
                        case uint8('c')
                            tagCode = uint32(1);
                        case uint8('d')
                            tagCode = uint32(2);
                        case uint8('g')
                            tagCode = uint32(3);
                        case uint8('n')
                            tagCode = uint32(4);
                        case uint8('r')
                            tagCode = uint32(5);
                        case uint8('s')
                            tagCode = uint32(6);
                        case uint8('t')
                            tagCode = uint32(7);
                    end
                    if(tagCode)
                        tagMode = uint32(1);
                    end
                case uint32(1) % one character: ':'
                    if(uint8(':') == bytes(i))
                        tagMode = uint32(2);
                        L = uint32(1);
                    else
                        tagMode = uint32(0);
                    end
                case uint32(2) % several characters up to next ',' or '*'
                    if(uint8(',') == bytes(i))
                        tagMode = uint32(0);
                    elseif(uint8('*') == bytes(i))
                        tagMode = uint32(3);
                    elseif(tagCode && (L <= 16))
                        TAGbuffer(L, tagCode) = uint8(bytes(i));
                        L = L + uint32(1);
                    end
                case uint32(3) % one character: MSB of checksum
                    strCS(1) = bytes(i);
                    tagMode = uint32(4);
                case uint32(4) % one character: LSB of checksum
                    strCS(2) = bytes(i);
                    tagMode = uint32(5);
                    if(~ignoreChecksum)
                        checksumCorrect = (cs == uint8(hex2dec(char(strCS))));
                    end
            end
            if(tagMode < uint32(3))
                cs = bitxor(cs,bytes(i));
            end
            continue;
        end

        % After the TAG block: payload
        if((tagMode >= uint32(5)) && checksumCorrect)
            payloadLength = payloadLength + uint32(1);
            payloadBytes(payloadLength) = bytes(i);
        end
    end

    % ~~~~~~~~~~~~~~~~~~~~~~~~~~~~~~~~~~~~~~~~~~~~~~~~~~~~~~~~~~~~~~~~~~~~~~~~~~~~~~~~~~~~~~~~~~~~~~~~~~~~~~~~~~~~~~~~~~~~~~~~~
    % Set TAG outputs
    % ~~~~~~~~~~~~~~~~~~~~~~~~~~~~~~~~~~~~~~~~~~~~~~~~~~~~~~~~~~~~~~~~~~~~~~~~~~~~~~~~~~~~~~~~~~~~~~~~~~~~~~~~~~~~~~~~~~~~~~~~~
    if(~checksumCorrect)
        TAGbuffer = uint8(zeros(16,7));
    end
    tag_c = TAGbuffer(:,1);
    tag_d = TAGbuffer(:,2);
    tag_g = TAGbuffer(:,3);
    tag_n = TAGbuffer(:,4);
    tag_r = TAGbuffer(:,5);
    tag_s = TAGbuffer(:,6);
    tag_t = TAGbuffer(:,7);
end

== matlab function NMEA/Encoder/NMEA 0183 Encode RMC/EncodeMagneticVariation ==
  data: magVar input double size=1; magVarDeg output double size=1; magVarChar output uint8 size=1
function [magVarDeg, magVarChar] = EncodeMagneticVariation(magVar)
    % Ensure that input angle is symmetric
    x = magVar;
    x = x - 6.28318530717959 * fix(x * 0.159154943091895);
    magVar = x + 6.28318530717959 * double(x < -3.14159265358979) - 6.28318530717959 * double(x >= 3.14159265358979);

    % Set character
    magVarChar = uint8('E');
    if(magVar < 0.0)
        magVarChar = uint8('W');
    end

    % Set angle in degrees
    magVarDeg = rad2deg(abs(magVar));
end

== matlab function NMEA/Details/Select NMEA and Fill Empty Fields/SelectMessageAndFillEmptyFields ==
  data: u input; y output
function y = SelectMessageAndFillEmptyFields(u)
    % Replace ",," by ",0," and replace ",*" by ",0*"
    N = 32 + length(u) - 8;
    y = uint8(zeros(N, 1));
    iy = 1;
    % Ignore first 8 bytes (timestamp) and start with byte 9
    for i = 9:length(u)
        if((i > 9) && (((uint8(',') == u(i)) || (uint8('*') == u(i))) && (uint8(',') == u(i-1))))
            y(iy) = uint8('0');
            iy = iy + 1;
            if(iy > N), break; end
        end
        y(iy) = u(i);
        iy = iy + 1;
        if(iy > N), break; end
    end
end

== matlab function NMEA/Decoder/NMEA 0183 Decode MWV/DecodeMessage/MATLAB Function ==
  data: windSpeedValue input double size=1; windSpeed output double size=1; windSpeedUnit input uint8 size=1
function windSpeed = fcn(windSpeedValue, windSpeedUnit)
    windSpeed = windSpeedValue;
    if((uint8('K') == windSpeedUnit) || (uint8('k') == windSpeedUnit))
        % km/h to m/s
        windSpeed = windSpeedValue / 3.6;
    elseif((uint8('N') == windSpeedUnit) || (uint8('n') == windSpeedUnit))
        % knots to m/s
        windSpeed = windSpeedValue * 0.51444444444444444;
    end
end
